simulink model "sra2_1"  (R2016a)
settings: Solver=ode45  StartTime=0  StopTime=30  RelTol=1e-5
values from neighbouring files (symbols this model uses):
  a1 = 0    [program2.m]    (also in program3.m = Hpcd.den{1}(2))
  a2 = 6.23    [program2.m]
  b = -291.8    [program2.m]    (also in program3.m = Hpcd.num{1}(3)/Hpcd.num{1}(2))
  c = 6    [program2.m]
  delta = 0.1    [program2.m]
  ftilda = 1000    [program2.m]
  Ti = 0.1605    [program2.m]
libraries: simulink x1
settings Model: Creator=andrei  LastModifiedBy=andrei

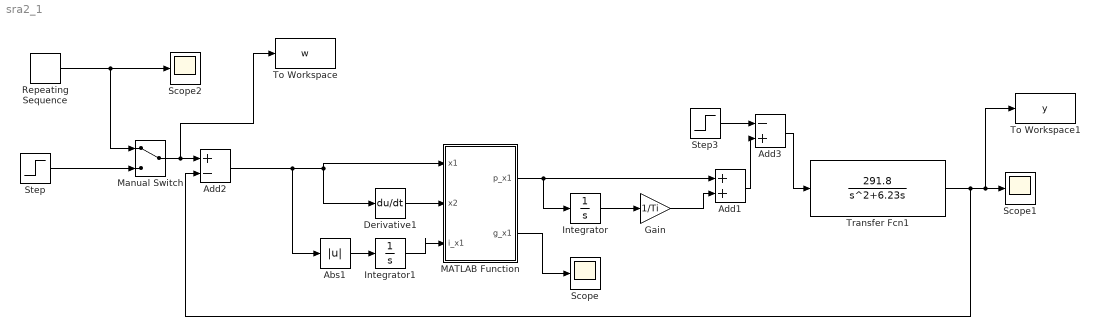
== system sra2_1 ==
  Abs1 : Abs
  Add1 : Sum
  Add2 : Sum  Inputs=+-
  Add3 : Sum  Inputs=-+
  Derivative1 : Derivative
  Gain : Gain  Gain=1/Ti
  Integrator : Integrator
  Integrator1 : Integrator
  MATLAB Function : MATLAB Function  TreatAsAtomicUnit=on
  Manual Switch : ManualSwitch
  Repeating Sequence : simulink/Sources/Repeating Sequence  rep_seq_t=[0.0001 5 5.0001 10 10.0001]  rep_seq_y=[0.0001 0.0000 5 5 5]
  Scope : Scope
  Scope1 : Scope
  Scope2 : Scope
  Step : Step  Time=0  SampleTime=0
  Step3 : Step  Time=7.5  After=0.01  SampleTime=0
  To Workspace : ToWorkspace  VariableName=w  SaveFormat=Timeseries  SampleTime=-1
  To Workspace1 : ToWorkspace  VariableName=y  SaveFormat=Timeseries  SampleTime=-1
  Transfer Fcn1 : TransferFcn  Numerator=[291.8]  Denominator=[1 6.23 0]
  wires:
  MATLAB Function/2(g_x1) -> Scope/1
  Integrator/1 -> Gain/1
  Gain/1 -> Add1/2
  MATLAB Function/1(p_x1) -> Integrator/1, Add1/1
  Integrator1/1 -> MATLAB Function/3(i_x1)
  Abs1/1 -> Integrator1/1
  Derivative1/1 -> MATLAB Function/2(x2)
  Add2/1 -> Abs1/1, Derivative1/1, MATLAB Function/1(x1)
  Transfer Fcn1/1 -> Add2/2, To Workspace1/1, Scope1/1
  Repeating Sequence/1 -> Manual Switch/1, Scope2/1
  Step/1 -> Manual Switch/2
  Manual Switch/1 -> To Workspace/1, Add2/1
  Add3/1 -> Transfer Fcn1/1
  Step3/1 -> Add3/1
  Add1/1 -> Add3/2

== matlab function sra2_1/MATLAB Function ==
  data: x1 input; p_x1 output; x2 input; i_x1 input; g_x1 output; c parameter; a1 parameter; a2 parameter; ftilda parameter; delta parameter; b parameter; Ti parameter
function [p_x1,g_x1] = fcn(x1,x2,i_x1,c, a1, a2, ftilda, delta, b, Ti)

alfa=(abs((c^2-a2*c+a1)*x1)+ftilda)/(abs(b)*abs(x1)+1/Ti*i_x1)+delta;

g_x1=(c*x1+x2)*x1;

p_x1=alfa*sign(g_x1)*x1;

end
